simulink model "final_quadruped_080622_vel_level control"  (R2021a)
settings: Solver=ode15s  StartTime=0.0  StopTime=10  RelTol=1e-3  EnableMultiTasking=on
values from neighbouring files (symbols this model uses):
  foot_x = 8    [bipedparameters.m]    (also in fcn.m; finalrobotParameters.m; finalrobotParameters_110522.m; finalrobotParameters_140522.m)
  foot_y = 6    [bipedparameters.m]    (also in fcn.m; finalrobotParameters.m; finalrobotParameters_110522.m; finalrobotParameters_140522.m)
  foot_z = 1    [bipedparameters.m]    (also in fcn.m; finalrobotParameters.m; finalrobotParameters_110522.m; finalrobotParameters_140522.m)
  height_plane = 0.025    [bipedparameters.m]    (also in finalrobotParameters.m; finalrobotParameters_110522.m; finalrobotParameters_140522.m; finalrobotParameters_240522.m)
  kd = 1000    [bipedparameters.m]    (also in finalrobotParameters_140522.m = 5; finalrobotParameters_240522.m)
  ki = 1000    [bipedparameters.m]    (also in finalrobotParameters_140522.m = 5; finalrobotParameters_240522.m)
  kp = 1000    [bipedparameters.m]    (also in finalrobotParameters_140522.m = 5; finalrobotParameters_240522.m)
  lower_leg_length = 10    [bipedparameters.m]    (also in fcn.m; finalrobotParameters.m; finalrobotParameters_110522.m; finalrobotParameters_140522.m)
  m_ll = density*leg_radius*leg_radius*lower_leg_length*3.141592653589*0.01*0.01*0.01    (= 0.0176714586764)    [bipedparameters.m]    (also in fcn.m; finalrobotParameters_140522.m; finalrobotParameters_240522.m; hdotlb.m)
  m_ul = density*leg_radius*leg_radius*upper_leg_length*3.141592653589*0.01*0.01*0.01    (= 0.0176714586764)    [bipedparameters.m]    (also in fcn.m; finalrobotParameters_140522.m; finalrobotParameters_240522.m; hdotlb.m)
  plane_x = 25    [bipedparameters.m]    (also in finalrobotParameters.m; finalrobotParameters_110522.m; finalrobotParameters_140522.m; finalrobotParameters_240522.m)
  plane_y = 3    [bipedparameters.m]    (also in finalrobotParameters.m; finalrobotParameters_110522.m; finalrobotParameters_140522.m; finalrobotParameters_240522.m)
  torso_offset_x = -0.5    [bipedparameters.m]    (also in finalrobotParameters.m = 10; finalrobotParameters_110522.m = 10; finalrobotParameters_140522.m = 10; finalrobotParameters_240522.m = 10)
  torso_offset_z = -2    [bipedparameters.m]    (also in finalrobotParameters.m; finalrobotParameters_110522.m; finalrobotParameters_140522.m; finalrobotParameters_240522.m)
  torso_x = 5    [bipedparameters.m]    (also in fcn.m = 25; finalrobotParameters.m = 25; finalrobotParameters_110522.m = 25; finalrobotParameters_140522.m = 25)
  torso_y = 10    [bipedparameters.m]    (also in fcn.m = 16; finalrobotParameters.m = 16; finalrobotParameters_110522.m = 16; finalrobotParameters_140522.m = 16)
  torso_z = 8    [bipedparameters.m]    (also in fcn.m = 10; finalrobotParameters.m = 10; finalrobotParameters_110522.m = 10; finalrobotParameters_140522.m = 10)
  upper_leg_length = 10    [bipedparameters.m]    (also in fcn.m; finalrobotParameters.m; finalrobotParameters_110522.m; finalrobotParameters_140522.m)
undefined symbols (not defined in the file or in its folder): angleLFknee, speedLFknee, torqueLFknee, X, Y, Z
libraries: nesl_utility x105, sm_lib x71, Contact_Forces_Lib x16, pid_lib x12, fl_lib x3
(part 1 of 6)
settings Model: Creator=Durbadal Guest  LastModifiedBy=Saniya
settings SolverCC: AlgebraicLoopSolver=TrustRegion
settings DataIOCC: LimitDataPoints=on  SaveFormat=StructureWithTime  ReturnWorkspaceOutputs=off
settings OptimizationCC: LifeSpan=inf
settings DebuggingCC: SFUnexpectedBacktrackingDiag=warning  SFNoUnconditionalDefaultTransitionDiag=warning  SFExecutionAtInitializationDiag=none  SFMachineParentedDataDiag=warning  ArithmeticOperatorsInVariantConditions=warning
settings HardwareCC: ProdBitPerSizeT=32  ProdBitPerPtrDiffT=32  ProdWordSize=32  ProdHWDeviceType=Specified
settings SFSimCC: SimUseLocalCustomCode=off  CustomCodeUndefinedFunction=UseInterfaceOnly
settings RTWCC: RTWUseLocalCustomCode=off
settings CodeAppCC: StateflowObjectComments=on
settings GRTTargetCC: TargetLangStandard=C89/C90 (ANSI)
settings ConfigComp: CovMetricSettings=dw  CovSaveCumulativeToWorkspaceVar=on  CovSaveSingleToWorkspaceVar=on  CovExternalEMLEnable=off  CovSFcnEnable=off
settings SimscapeCC: SimscapeNominalValues="[{\"value\":\"10\",\"unit\":\"V\"},{\"value\":\"1\",\"unit\":\"A\"},{\"value\":\"10\",\"unit\":\"N*m\"},{\"value\":\"10\",\"unit\":\"bar\"},{\"value\":\"100\",\"unit\":\"kJ/kg\"},{\"value\":\"1\",\"unit\":\"kW\"},{\"value\":\"300\",\"unit\":\"K\"},{\"value\":\"100\",\"unit\":\"cm^3/s\"},{\"value\":\"1\",\"unit\":\"kN\"},{\"value\":\"1\",\"unit\":\"g/cm^3\"},{\"value\":\"1\",\"unit\":\"l\"},{\"value\":\"1\",\"unit\":\"cm^2\"},{\"value\":\"60\",\"unit\":\"Hz\"}]"  SimscapeLogType=all  SimscapeLogDataHistory=10000
settings ConfigurationSet: Description=SimMechanics 2G
settings DiagnosticsConfigSet: SimMechanicsRigidlyBoundBlock=none

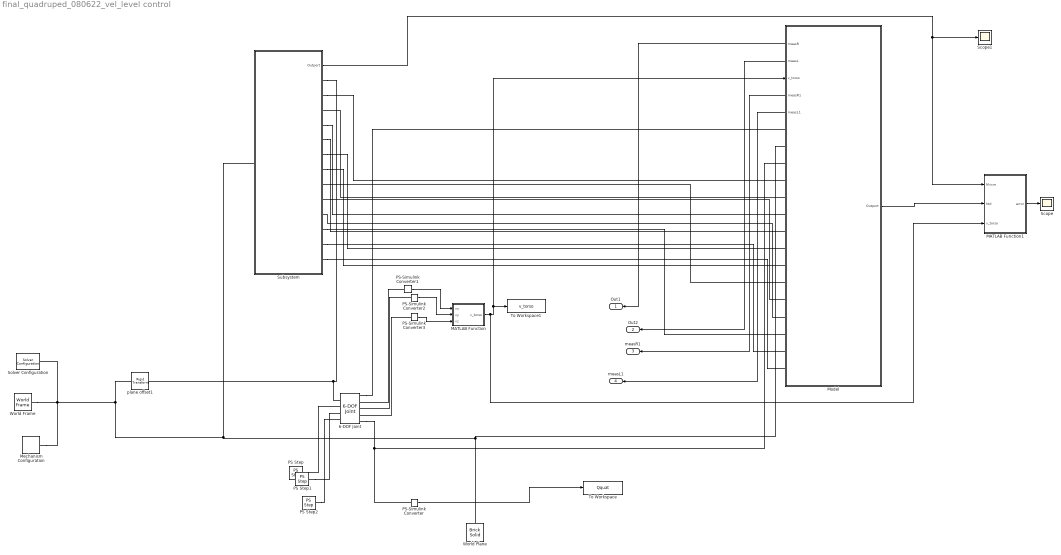
== system final_quadruped_080622_vel_level control ==
  6-DOF Joint : sm_lib/Joints/6-DOF Joint  JointMode=Normal  SenseConstraintForce=off  SenseConstraintForceX=off  SenseConstraintForceY=off  SenseConstraintForceZ=off  SenseConstraintTorque=off  SenseConstraintTorqueX=off  SenseConstraintTorqueY=off  SenseConstraintTorqueZ=off  SenseTotalForce=off  SenseTotalForceX=off  SenseTotalForceY=off  SenseTotalForceZ=off  SenseTotalTorque=off  SenseTotalTorqueX=off  SenseTotalTorqueY=off  SenseTotalTorqueZ=off  CompositeWrenchDir=FollowerOnBase  CompositeWrenchFrame=BaseFrame  PxEquilibriumPosition=0  PxEquilibriumPositionUnits=m  PxSpringStiffness=0  PxSpringStiffnessUnits=N/m  PxDampingCoefficient=0  PxDampingCoefficientUnits=N/(m/s)  PxTorqueActuationMode=InputTorque  PxMotionActuationMode=ComputedMotion  PxSensePosition=off  PxSenseVelocity=on  PxSenseAcceleration=off  PxSenseTorqueForce=off  PxSenseLowerLimitTorqueForce=off  PxSenseUpperLimitTorqueForce=off  PxLowerLimitSpecify=off  PxLowerLimitBound=-1  PxLowerLimitBoundUnits=m  PxLowerLimitStiffness=1e6  PxLowerLimitStiffnessUnits=N/m  PxLowerLimitDamping=1e3  PxLowerLimitDampingUnits=N/(m/s)  PxLowerLimitTransitionRegionWidth=1e-4  PxLowerLimitTransitionRegionWidthUnits=m  PxUpperLimitSpecify=off  PxUpperLimitBound=1  PxUpperLimitBoundUnits=m  PxUpperLimitStiffness=1e6  PxUpperLimitStiffnessUnits=N/m  PxUpperLimitDamping=1e3  PxUpperLimitDampingUnits=N/(m/s)  PxUpperLimitTransitionRegionWidth=1e-4  PxUpperLimitTransitionRegionWidthUnits=m  PxPositionTargetSpecify=on  PxPositionTargetPriority=High  PxPositionTargetValue=0  PxPositionTargetValueUnits=m  PxVelocityTargetSpecify=off  PxVelocityTargetPriority=High  PxVelocityTargetValue=0  PxVelocityTargetValueUnits=m/s  PyEquilibriumPosition=0  PyEquilibriumPositionUnits=m  PySpringStiffness=0  PySpringStiffnessUnits=N/m  PyDampingCoefficient=0  PyDampingCoefficientUnits=N/(m/s)  PyTorqueActuationMode=InputTorque  PyMotionActuationMode=ComputedMotion  PySensePosition=off  PySenseVelocity=on  PySenseAcceleration=off  PySenseTorqueForce=off  PySenseLowerLimitTorqueForce=off  PySenseUpperLimitTorqueForce=off  PyLowerLimitSpecify=off  PyLowerLimitBound=-1  PyLowerLimitBoundUnits=m  PyLowerLimitStiffness=1e6  PyLowerLimitStiffnessUnits=N/m  PyLowerLimitDamping=1e3  PyLowerLimitDampingUnits=N/(m/s)  PyLowerLimitTransitionRegionWidth=1e-4  PyLowerLimitTransitionRegionWidthUnits=m  PyUpperLimitSpecify=off  PyUpperLimitBound=1  PyUpperLimitBoundUnits=m  PyUpperLimitStiffness=1e6  PyUpperLimitStiffnessUnits=N/m  PyUpperLimitDamping=1e3  PyUpperLimitDampingUnits=N/(m/s)  PyUpperLimitTransitionRegionWidth=1e-4  PyUpperLimitTransitionRegionWidthUnits=m  PyPositionTargetSpecify=on  PyPositionTargetPriority=High  PyPositionTargetValue=0  PyPositionTargetValueUnits=m  PyVelocityTargetSpecify=off  PyVelocityTargetPriority=High  PyVelocityTargetValue=0  PyVelocityTargetValueUnits=m/s  PzEquilibriumPosition=0  PzEquilibriumPositionUnits=m  PzSpringStiffness=0  PzSpringStiffnessUnits=N/m  PzDampingCoefficient=0  PzDampingCoefficientUnits=N/(m/s)  PzTorqueActuationMode=InputTorque  PzMotionActuationMode=ComputedMotion  PzSensePosition=off  PzSenseVelocity=on  PzSenseAcceleration=off  PzSenseTorqueForce=off  PzSenseLowerLimitTorqueForce=off  PzSenseUpperLimitTorqueForce=off  PzLowerLimitSpecify=off  PzLowerLimitBound=-1  PzLowerLimitBoundUnits=m  PzLowerLimitStiffness=1e6  PzLowerLimitStiffnessUnits=N/m  PzLowerLimitDamping=1e3  PzLowerLimitDampingUnits=N/(m/s)  PzLowerLimitTransitionRegionWidth=1e-4  PzLowerLimitTransitionRegionWidthUnits=m  PzUpperLimitSpecify=off  PzUpperLimitBound=1  PzUpperLimitBoundUnits=m  PzUpperLimitStiffness=1e6  PzUpperLimitStiffnessUnits=N/m  PzUpperLimitDamping=1e3  PzUpperLimitDampingUnits=N/(m/s)  PzUpperLimitTransitionRegionWidth=1e-4  PzUpperLimitTransitionRegionWidthUnits=m  PzPositionTargetSpecify=on  PzPositionTargetPriority=High  PzPositionTargetValue=0  PzPositionTargetValueUnits=m  PzVelocityTargetSpecify=off  PzVelocityTargetPriority=High  PzVelocityTargetValue=0  PzVelocityTargetValueUnits=m/s  SphDefPosRotationMethod=None  SphDefPosRotationAngleUnits=deg  SphDefPosRotationStandardAxis=+Z  SphDefPosRotationAngle=0.0  SphDefPosRotationArbitraryAxis=[0 0 1]  SphDefPosFollAlignAxisA=+X  SphDefPosBaseAlignAxisA=+Y  SphDefPosFollAlignAxisB=+Y  SphDefPosBaseAlignAxisB=+Z  SphDefPosRotationSequenceAxes=FollowerAxes  SphDefPosRotationSequence=XYX  SphDefPosRotationSequenceAngles=[0 0 0]  SphDefPosRotationSequenceAnglesUnits=deg  SphDefPosRotationMatrix=[1 0 0; 0 1 0; 0 0 1]  SphEqPosRotationMethod=None  SphEqPosRotationAngleUnits=deg  SphEqPosRotationStandardAxis=+Z  SphEqPosRotationAngle=0.0  SphEqPosRotationArbitraryAxis=[0 0 1]  SphEqPosFollAlignAxisA=+X  SphEqPosBaseAlignAxisA=+Y  SphEqPosFollAlignAxisB=+Y  SphEqPosBaseAlignAxisB=+Z  SphEqPosRotationSequenceAxes=FollowerAxes  SphEqPosRotationSequence=XYX  SphEqPosRotationSequenceAngles=[0 0 0]  SphEqPosRotationSequenceAnglesUnits=deg  SphEqPosRotationMatrix=[1 0 0; 0 1 0; 0 0 1]  SphSpringStiffness=0  SphSpringStiffnessUnits=N*m/deg  SphDampingCoefficient=world_rot_damping  SphDampingCoefficientUnits=N*m/(deg/s)  SphActuateTorqueX=off  SphActuateTorqueY=off  SphActuateTorqueZ=off  SphActuateTorque=off  SphTorqueActuationMode=NoTorque  SphMotionActuationMode=ComputedMotion  SphActuationFrame=BaseFrame  SphSensePosition=on  SphSenseVelocityX=off  SphSenseVelocityY=off  SphSenseVelocityZ=off  SphSenseVelocity=off  SphSenseAccelerationX=off  SphSenseAccelerationY=off  SphSenseAccelerationZ=off  SphSenseAcceleration=off  SphSenseTorqueX=off  SphSenseTorqueY=off  SphSenseTorqueZ=off  SphSenseTorqueForce=off  SphSenseLowerLimitTorqueMag=off  SphSenseUpperLimitTorqueMag=off  SphSensingFrame=BaseFrame  SphLowerLimitSpecify=off  SphLowerLimitBound=15  SphLowerLimitBoundUnits=deg  SphLowerLimitStiffness=1e4  SphLowerLimitStiffnessUnits=N*m/deg  SphLowerLimitDamping=10  SphLowerLimitDampingUnits=N*m/(deg/s)  SphLowerLimitTransitionRegionWidth=0.1  SphLowerLimitTransitionRegionWidthUnits=deg  SphUpperLimitSpecify=off  SphUpperLimitBound=45  SphUpperLimitBoundUnits=deg  SphUpperLimitStiffness=1e4  SphUpperLimitStiffnessUnits=N*m/deg  SphUpperLimitDamping=10  SphUpperLimitDampingUnits=N*m/(deg/s)  SphUpperLimitTransitionRegionWidth=0.1  SphUpperLimitTransitionRegionWidthUnits=deg  SphPositionTargetRotationMethod=None  SphPositionTargetRotationAngleUnits=deg  SphPositionTargetRotationStandardAxis=+Z  SphPositionTargetRotationAngle=0.0  SphPositionTargetRotationArbitraryAxis=[0 0 1]  SphPositionTargetFollAlignAxisA=+X  SphPositionTargetBaseAlignAxisA=+Y  SphPositionTargetFollAlignAxisB=+Y  SphPositionTargetBaseAlignAxisB=+Z  SphPositionTargetRotationSequenceAxes=FollowerAxes  SphPositionTargetRotationSequence=XYX  SphPositionTargetRotationSequenceAngles=[0 0 0]  SphPositionTargetRotationSequenceAnglesUnits=deg  SphPositionTargetRotationMatrix=[1 0 0; 0 1 0; 0 0 1]  SphPositionTargetSpecify=off  SphPositionTargetPriority=High  SphVelocityTargetValue=[0 0 0]  SphVelocityTargetValueUnits=deg/s  SphVelocityTargetSpecify=off  SphVelocityTargetPriority=High  SphVelocityTargetInFollowerFrame=on
  MATLAB Function : MATLAB Function  TreatAsAtomicUnit=on
  MATLAB Function1 : MATLAB Function  TreatAsAtomicUnit=on
  Mechanism Configuration : sm_lib/Utilities/Mechanism Configuration  UniformGravity=Constant  GravityVector=[0 0 -9.80665]  GravityVectorUnits=m/s^2  GravityUnits=m/s^2  LinearizationDelta=0.001  JointModeTransitionNonlinearIterations=2
  Model : Subsystem
      settings: PortSchema="{\"entries\":[{\"content\":{\"sides\":[{\"content\":{\"connectorIds\":[\"Out5\"]},\"type\":\"ConnectorPlacement.EquallySpacedRectSide\",\"uuid\":\"648e0f1c-94fd-432d-b314-f859853b28dc\"},{\"content\":{\"connectorIds\":[\"Out1\",\"Out2\",\"In1\",\"Out3\",\"Out4\",\"RConn1\",\"RConn2\",\"RConn3\",\"RConn4\",\"RConn5\",\"RConn6\",\"RConn7\",\"RConn8\",\"RConn9\",\"RConn10\",\"RConn11\",\"RConn12\",\"RConn13\",\"RConn14\",\"RConn15\"],\"side\":\"RIGHT\"},\"type\":\"ConnectorPlacement.EquallySpacedRectSide\",\"uuid\":\"4a085109-6c7b-452e-9c34-33db191f9143\"},{\"content\":{\"connectorIds\":[],\"side\":\"TOP\"},\"type\":\"ConnectorPlacement.EquallySpacedRectSide\",\"uuid\":\"a578f37e-fb06-4d5d-8e21-8bc1ba433708\"}]},\"type\":\"ConnectorPlacement.EquallySpacedConnector\",\"uuid\":\"512c293d-fddc-4597-a716-0ff05cc0aa2f\"}],\"packageUris\":[\"http://schema.mathworks.com/mf0/Connector/R2020b\"],\"version\":\"1.0\"}"
  PS Step : fl_lib/Physical Signals/Sources/PS Step  step_time=0 s  initial_value=0 N  final_value=1 N
      settings: SourceProductBaseCode=SS
  PS Step1 : fl_lib/Physical Signals/Sources/PS Step  step_time=0 s  initial_value=0 N  final_value=0 N
      settings: SourceProductBaseCode=SS
  PS Step2 : fl_lib/Physical Signals/Sources/PS Step  step_time=0 s  initial_value=0 N  final_value=5 N
      settings: SourceProductBaseCode=SS
  PS-Simulink Converter{,1..3} (4 alike) : nesl_utility/PS-Simulink Converter  PhysicalDomain=network_engine_domain  SubClassName=ps_output  LeftPortType=input  RightPortType=output  PseudoPeriodic=off  Frequencies=[]  Unit=inherit  AffineConversion=off
      settings: SourceProductBaseCode=PW,SS
  Scope : Scope
  Scope1 : Scope
  Solver Configuration : nesl_utility/Solver Configuration  PhysicalDomain=network_engine_domain  SubClassName=solver  LeftPortType=input  RightPortType=generic  Tones=[]  Harmonics=[]  SimulateNoise=off  Profile=off  UseLocalSampling=off  EnableSwitchedLinearOptims=on  FrequencyDomain=off  UseCCode=off  RelTol=0.001  AbsTol=1e-06  MinStep=1e-09  ToWorkspace=off  RevertToSquareIcSolve=off  NumHomotopyIterations=100  PhasorMode=off  PhasorModeNumHarmonics=1  DoDC=off  ResidualTolerance=1e-09  UseLocalSolver=off  LocalSolverChoice=NE_BACKWARD_EULER_ADVANCER  LocalSolverSampleTime=0.001  DoFixedCost=off  MaxNonlinIter=3  MaxModeIter=2  ComputeImpulses=off  ImpulseIterations=2  LinearAlgebra=Full  EquationFormulation=NE_TIME_EF  DelaysMemoryBudget=1024  AutomaticFiltering=on  FilteringTimeConstant=0.001  PartitionStorageMethod=AS_NEEDED  PartitionMemoryBudget=1024  PartitionMethod=FAST
      settings: SourceProductBaseCode=PW,SS
  Subsystem : Subsystem
  To Workspace : ToWorkspace  VariableName=Qquat  SaveFormat=Timeseries  SampleTime=-1
  To Workspace1 : ToWorkspace  VariableName=v_torso  SaveFormat=Timeseries  SampleTime=-1
  World Frame : sm_lib/Frames and Transforms/World Frame
  World Plane : sm_lib/Body Elements/Brick Solid  GraphicAmbientColor=[0.15 0.15 0.15 1.0]  BasedOnType=Density  BrickDimensions=[plane_x plane_y height_plane]  BrickDimensionUnits=m  CenterOfMass=[0 0 0]  CenterOfMassUnits=m  GraphicDiffuseColor=[1.0 0.2 0.2]  Density=2000  DensityUnits=kg/m^3  DoExposeReferenceFrame=on  GraphicEmissiveColor=[0.0 0.0 0.0 1.0]  ExportEntireGeometry=off  SerializedFrames=<Frames/>  MarkerShape=Sphere  MarkerSize=10  GraphicType=FromGeometry  InertiaType=CalculateFromGeometry  Mass=1  MassUnits=kg  MomentsOfInertia=[1 1 1]  MomentsOfInertiaUnits=kg*m^2  GraphicOpacity=1.0  ProductsOfInertia=[1 1 1]  ProductsOfInertiaUnits=kg*m^2  GraphicShininess=75  GraphicSpecularColor=[0.5 0.5 0.5 1.0]  GraphicVisPropType=SimpleVisualProperties
  plane offset1 : sm_lib/Frames and Transforms/Rigid Transform  TranslationMethod=StandardAxis  TranslationStandardOffset=24.1  TranslationLengthUnit=cm  TranslationStandardAxis=+Z  TranslationCartesianOffset=[0 0 0]  TranslationROffset=0  TranslationROffsetUnits=m  TranslationZOffset=0  TranslationZOffsetUnits=m  TranslationThetaOffset=0  TranslationThetaOffsetUnits=deg  RotationMethod=None  RotationAngleUnits=deg  RotationStandardAxis=+Z  RotationAngle=0.0  RotationArbitraryAxis=[0 0 1]  FollAlignAxisA=+X  BaseAlignAxisA=+Y  FollAlignAxisB=+Y  BaseAlignAxisB=+Z  RotationSequenceAxes=FollowerAxes  RotationSequence=XYX  RotationSequenceAngles=[0 0 0]  RotationSequenceAnglesUnits=deg  RotationMatrix=[1 0 0; 0 1 0; 0 0 1]
  Out1 : Outport  VectorParamsAs1DForOutWhenUnconnected=off
  Out2 : Outport  Port=2  VectorParamsAs1DForOutWhenUnconnected=off
  measR1 : Outport  Port=3  VectorParamsAs1DForOutWhenUnconnected=off
  measL1 : Outport  Port=4  VectorParamsAs1DForOutWhenUnconnected=off
  wires:
  Model/1(measR) -> Out1/1
  Model/2(measL) -> Out2/1
  Model/3(measR1) -> measR1/1
  Model/4(measL1) -> measL1/1
  PS-Simulink Converter/1 -> To Workspace/1
  PS-Simulink Converter1/1 -> MATLAB Function/1(vx)
  PS-Simulink Converter2/1 -> MATLAB Function/2(vy)
  PS-Simulink Converter3/1 -> MATLAB Function/3(vz)
  MATLAB Function/1(v_torso) -> MATLAB Function1/3(v_torso), To Workspace1/1, Model/1(v_torso)
  Subsystem/1(Outport) -> Scope1/1, MATLAB Function1/1(Mvcm)
  Model/5(Outport) -> MATLAB Function1/2(htd)
  MATLAB Function1/1(error) -> Scope/1
  connections:
  6-DOF Joint/RConn1 -- Model/RConn1
  6-DOF Joint/LConn1 -- plane offset1/RConn1 -- Subsystem/RConn1
  6-DOF Joint/RConn5 -- PS-Simulink Converter/LConn1 -- Model/RConn3
  PS-Simulink Converter1/LConn1 -- 6-DOF Joint/RConn2
  PS-Simulink Converter2/LConn1 -- 6-DOF Joint/RConn3
  PS-Simulink Converter3/LConn1 -- 6-DOF Joint/RConn4
  plane offset1/LConn1 -- Solver Configuration/RConn1 -- World Frame/RConn1 -- Mechanism Configuration/RConn1 -- World Plane/RConn1 -- Model/RConn2 -- Subsystem/LConn1
  Subsystem/RConn2 -- Model/RConn4
  Model/RConn5 -- Subsystem/RConn3
  Subsystem/RConn4 -- Model/RConn6
  Subsystem/RConn5 -- Model/RConn7
  Subsystem/RConn6 -- Model/RConn8
  Subsystem/RConn7 -- Model/RConn9
  Model/RConn10 -- Subsystem/RConn8
  Model/RConn11 -- Subsystem/RConn9
  Model/RConn12 -- Subsystem/RConn10
  Subsystem/RConn11 -- Model/RConn13
  Subsystem/RConn12 -- Model/RConn14
  Subsystem/RConn13 -- Model/RConn15
  6-DOF Joint/LConn2 -- PS Step/RConn1
  PS Step1/RConn1 -- 6-DOF Joint/LConn3
  PS Step2/RConn1 -- 6-DOF Joint/LConn4

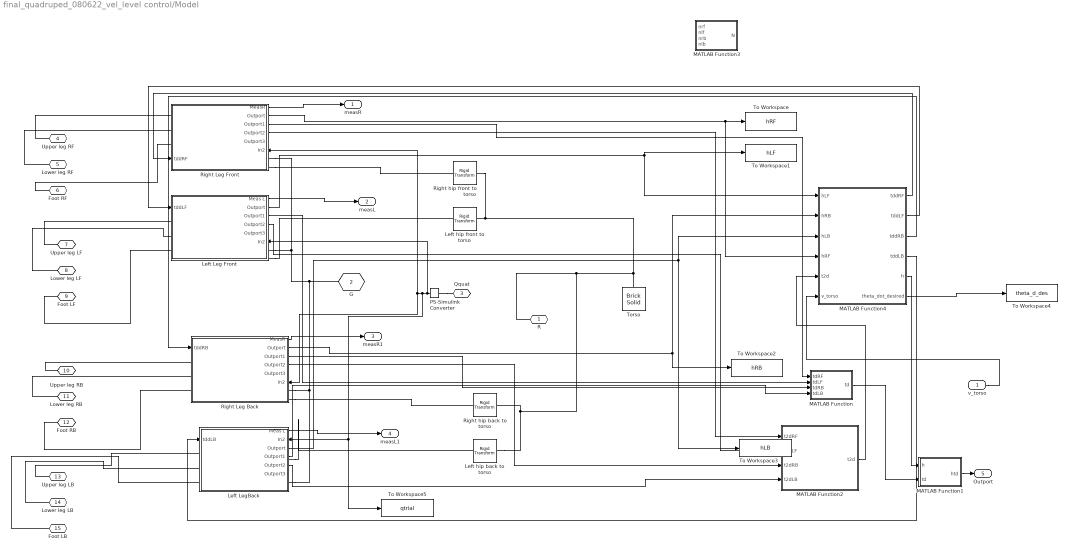
== system final_quadruped_080622_vel_level control/Model ==
  v_torso : Inport
  Left Leg Front : Subsystem
      settings: PortSchema="{\"entries\":[{\"content\":{\"sides\":[{\"content\":{\"connectorIds\":[\"In1\",\"LConn1\",\"LConn2\",\"LConn3\"]},\"type\":\"ConnectorPlacement.EquallySpacedRectSide\",\"uuid\":\"1507813e-36a9-49af-9b0a-e3846bbe4283\"},{\"content\":{\"connectorIds\":[\"Out1\",\"Out2\",\"Out3\",\"Out4\",\"Out5\",\"In2\",\"RConn1\",\"RConn2\"],\"side\":\"RIGHT\"},\"type\":\"ConnectorPlacement.EquallySpacedRectSide\",\"uuid\":\"5066f35d-c1fd-4314-a197-bec554758284\"},{\"content\":{\"connectorIds\":[],\"side\":\"TOP\"},\"type\":\"ConnectorPlacement.EquallySpacedRectSide\",\"uuid\":\"2e06378b-9fb7-4b7b-9b3c-942eabd1dde3\"}]},\"type\":\"ConnectorPlacement.EquallySpacedConnector\",\"uuid\":\"ce1b660b-7838-4ff4-b715-b13e7b6fd161\"}],\"packageUris\":[\"http://schema.mathworks.com/mf0/Connector/R2020b\"],\"version\":\"1.0\"}"
  Left LegBack : Subsystem
      settings: PortSchema="{\"entries\":[{\"content\":{\"sides\":[{\"content\":{\"connectorIds\":[\"In1\",\"LConn1\",\"LConn2\",\"LConn3\"]},\"type\":\"ConnectorPlacement.EquallySpacedRectSide\",\"uuid\":\"22ee734e-d516-4767-9dd7-a84a6d7499a1\"},{\"content\":{\"connectorIds\":[\"Out1\",\"In2\",\"Out2\",\"Out3\",\"Out4\",\"Out5\",\"RConn1\",\"RConn2\"],\"side\":\"RIGHT\"},\"type\":\"ConnectorPlacement.EquallySpacedRectSide\",\"uuid\":\"10c942f7-94ea-46a3-ba7f-65e81ae36ff4\"},{\"content\":{\"connectorIds\":[],\"side\":\"TOP\"},\"type\":\"ConnectorPlacement.EquallySpacedRectSide\",\"uuid\":\"f15406a8-c456-4a24-8e06-fd295582a32c\"}]},\"type\":\"ConnectorPlacement.EquallySpacedConnector\",\"uuid\":\"8882591f-f267-4868-b883-a2707b6c50ed\"}],\"packageUris\":[\"http://schema.mathworks.com/mf0/Connector/R2020b\"],\"version\":\"1.0\"}"
  Left hip back to torso : sm_lib/Frames and Transforms/Rigid Transform  TranslationMethod=Cartesian  TranslationStandardOffset=0  TranslationLengthUnit=cm  TranslationStandardAxis=+Z  TranslationCartesianOffset=[-torso_offset_x torso_y/2 torso_offset_z]  TranslationROffset=0  TranslationROffsetUnits=m  TranslationZOffset=0  TranslationZOffsetUnits=m  TranslationThetaOffset=0  TranslationThetaOffsetUnits=deg  RotationMethod=None  RotationAngleUnits=deg  RotationStandardAxis=+Z  RotationAngle=0.0  RotationArbitraryAxis=[0 0 1]  FollAlignAxisA=+X  BaseAlignAxisA=+Y  FollAlignAxisB=+Y  BaseAlignAxisB=+Z  RotationSequenceAxes=FollowerAxes  RotationSequence=XYX  RotationSequenceAngles=[0 0 0]  RotationSequenceAnglesUnits=deg  RotationMatrix=[1 0 0; 0 1 0; 0 0 1]
  Left hip front to torso : sm_lib/Frames and Transforms/Rigid Transform  TranslationMethod=Cartesian  TranslationStandardOffset=0  TranslationLengthUnit=cm  TranslationStandardAxis=+Z  TranslationCartesianOffset=[torso_offset_x torso_y/2 torso_offset_z]  TranslationROffset=0  TranslationROffsetUnits=m  TranslationZOffset=0  TranslationZOffsetUnits=m  TranslationThetaOffset=0  TranslationThetaOffsetUnits=deg  RotationMethod=None  RotationAngleUnits=deg  RotationStandardAxis=+Z  RotationAngle=0.0  RotationArbitraryAxis=[0 0 1]  FollAlignAxisA=+X  BaseAlignAxisA=+Y  FollAlignAxisB=+Y  BaseAlignAxisB=+Z  RotationSequenceAxes=FollowerAxes  RotationSequence=XYX  RotationSequenceAngles=[0 0 0]  RotationSequenceAnglesUnits=deg  RotationMatrix=[1 0 0; 0 1 0; 0 0 1]
  MATLAB Function : MATLAB Function  TreatAsAtomicUnit=on
  MATLAB Function1 : MATLAB Function  TreatAsAtomicUnit=on
  MATLAB Function2 : MATLAB Function  TreatAsAtomicUnit=on
  MATLAB Function3 : MATLAB Function  TreatAsAtomicUnit=on
  MATLAB Function4 : MATLAB Function  TreatAsAtomicUnit=on
  PS-Simulink Converter : nesl_utility/PS-Simulink Converter  PhysicalDomain=network_engine_domain  SubClassName=ps_output  LeftPortType=input  RightPortType=output  PseudoPeriodic=off  Frequencies=[]  Unit=inherit  AffineConversion=off
      settings: SourceProductBaseCode=PW,SS
  Right Leg Back : Subsystem
      settings: PortSchema="{\"entries\":[{\"content\":{\"sides\":[{\"content\":{\"connectorIds\":[\"In1\",\"LConn1\",\"LConn2\",\"LConn3\"]},\"type\":\"ConnectorPlacement.EquallySpacedRectSide\",\"uuid\":\"22ee734e-d516-4767-9dd7-a84a6d7499a1\"},{\"content\":{\"connectorIds\":[\"Out1\",\"Out2\",\"Out3\",\"Out4\",\"Out5\",\"In2\",\"RConn1\",\"RConn2\"],\"side\":\"RIGHT\"},\"type\":\"ConnectorPlacement.EquallySpacedRectSide\",\"uuid\":\"10c942f7-94ea-46a3-ba7f-65e81ae36ff4\"},{\"content\":{\"connectorIds\":[],\"side\":\"TOP\"},\"type\":\"ConnectorPlacement.EquallySpacedRectSide\",\"uuid\":\"f15406a8-c456-4a24-8e06-fd295582a32c\"}]},\"type\":\"ConnectorPlacement.EquallySpacedConnector\",\"uuid\":\"8882591f-f267-4868-b883-a2707b6c50ed\"}],\"packageUris\":[\"http://schema.mathworks.com/mf0/Connector/R2020b\"],\"version\":\"1.0\"}"
  "Right Leg Front " : Subsystem
      settings: PortSchema="{\"entries\":[{\"content\":{\"sides\":[{\"content\":{\"connectorIds\":[\"LConn1\",\"LConn2\",\"LConn3\",\"In1\"]},\"type\":\"ConnectorPlacement.EquallySpacedRectSide\",\"uuid\":\"22ee734e-d516-4767-9dd7-a84a6d7499a1\"},{\"content\":{\"connectorIds\":[\"Out1\",\"Out2\",\"Out3\",\"Out4\",\"Out5\",\"In2\",\"RConn1\",\"RConn2\"],\"side\":\"RIGHT\"},\"type\":\"ConnectorPlacement.EquallySpacedRectSide\",\"uuid\":\"10c942f7-94ea-46a3-ba7f-65e81ae36ff4\"},{\"content\":{\"connectorIds\":[],\"side\":\"TOP\"},\"type\":\"ConnectorPlacement.EquallySpacedRectSide\",\"uuid\":\"f15406a8-c456-4a24-8e06-fd295582a32c\"}]},\"type\":\"ConnectorPlacement.EquallySpacedConnector\",\"uuid\":\"8882591f-f267-4868-b883-a2707b6c50ed\"}],\"packageUris\":[\"http://schema.mathworks.com/mf0/Connector/R2020b\"],\"version\":\"1.0\"}"
  Right hip back to torso : sm_lib/Frames and Transforms/Rigid Transform  TranslationMethod=Cartesian  TranslationStandardOffset=0  TranslationLengthUnit=cm  TranslationStandardAxis=+Z  TranslationCartesianOffset=[-torso_offset_x -torso_y/2 torso_offset_z]  TranslationROffset=0  TranslationROffsetUnits=m  TranslationZOffset=0  TranslationZOffsetUnits=m  TranslationThetaOffset=0  TranslationThetaOffsetUnits=deg  RotationMethod=None  RotationAngleUnits=deg  RotationStandardAxis=+Z  RotationAngle=0.0  RotationArbitraryAxis=[0 0 1]  FollAlignAxisA=+X  BaseAlignAxisA=+Y  FollAlignAxisB=+Y  BaseAlignAxisB=+Z  RotationSequenceAxes=FollowerAxes  RotationSequence=XYX  RotationSequenceAngles=[0 0 0]  RotationSequenceAnglesUnits=deg  RotationMatrix=[1 0 0; 0 1 0; 0 0 1]
  Right hip front to torso : sm_lib/Frames and Transforms/Rigid Transform  TranslationMethod=Cartesian  TranslationStandardOffset=0  TranslationLengthUnit=cm  TranslationStandardAxis=+Z  TranslationCartesianOffset=[torso_offset_x -torso_y/2 torso_offset_z]  TranslationROffset=0  TranslationROffsetUnits=m  TranslationZOffset=0  TranslationZOffsetUnits=m  TranslationThetaOffset=0  TranslationThetaOffsetUnits=deg  RotationMethod=None  RotationAngleUnits=deg  RotationStandardAxis=+Z  RotationAngle=0.0  RotationArbitraryAxis=[0 0 1]  FollAlignAxisA=+X  BaseAlignAxisA=+Y  FollAlignAxisB=+Y  BaseAlignAxisB=+Z  RotationSequenceAxes=FollowerAxes  RotationSequence=XYX  RotationSequenceAngles=[0 0 0]  RotationSequenceAnglesUnits=deg  RotationMatrix=[1 0 0; 0 1 0; 0 0 1]
  To Workspace : ToWorkspace  VariableName=hRF  SaveFormat=Timeseries  SampleTime=-1
  To Workspace1 : ToWorkspace  VariableName=hLF  SaveFormat=Timeseries  SampleTime=-1
  To Workspace2 : ToWorkspace  VariableName=hRB  SaveFormat=Timeseries  SampleTime=-1
  To Workspace3 : ToWorkspace  VariableName=hLB  SaveFormat=Timeseries  SampleTime=-1
  To Workspace4 : ToWorkspace  VariableName=theta_d_des  SaveFormat=Timeseries  SampleTime=-1
  To Workspace5 : ToWorkspace  VariableName=qtrial  SaveFormat=Timeseries  SampleTime=-1
  Torso : sm_lib/Body Elements/Brick Solid  GraphicAmbientColor=[0.15 0.15 0.15 1.0]  BasedOnType=Density  BrickDimensions=[torso_x torso_y torso_z]  BrickDimensionUnits=cm  CenterOfMass=[0 0 0]  CenterOfMassUnits=m  GraphicDiffuseColor=[0.5 0.5 0.5]  Density=1000  DensityUnits=kg/m^3  DoExposeReferenceFrame=on  GraphicEmissiveColor=[0.0 0.0 0.0 1.0]  ExportEntireGeometry=off  SerializedFrames=<Frames/>  MarkerShape=Sphere  MarkerSize=10  GraphicType=FromGeometry  InertiaType=CalculateFromGeometry  Mass=1  MassUnits=kg  MomentsOfInertia=[1 1 1]  MomentsOfInertiaUnits=kg*m^2  GraphicOpacity=1.0  ProductsOfInertia=[1 1 1]  ProductsOfInertiaUnits=kg*m^2  GraphicShininess=75  GraphicSpecularColor=[0.5 0.5 0.5 1.0]  GraphicVisPropType=SimpleVisualProperties
  R : PMIOPort  Side=Right
  G : PMIOPort  Port=2  Side=Right
  Qquat : PMIOPort  Port=3  Side=Right
  Upper leg RF : PMIOPort  Port=4  Side=Right
  Lower leg RF : PMIOPort  Port=5  Side=Right
  Foot RF : PMIOPort  Port=6  Side=Right
  Upper leg LF : PMIOPort  Port=7  Side=Right
  Lower leg LF : PMIOPort  Port=8  Side=Right
  Foot LF : PMIOPort  Port=9  Side=Right
  Upper leg RB : PMIOPort  Port=10  Side=Right
  Lower leg RB : PMIOPort  Port=11  Side=Right
  Foot RB : PMIOPort  Port=12  Side=Right
  Upper leg LB : PMIOPort  Port=13  Side=Right
  Lower leg LB : PMIOPort  Port=14  Side=Right
  Foot LB : PMIOPort  Port=15  Side=Right
  measR : Outport  VectorParamsAs1DForOutWhenUnconnected=off
  measL : Outport  Port=2  VectorParamsAs1DForOutWhenUnconnected=off
  measR1 : Outport  Port=3  VectorParamsAs1DForOutWhenUnconnected=off
  measL1 : Outport  Port=4  VectorParamsAs1DForOutWhenUnconnected=off
  Outport : Outport  Port=5
  wires:
  Left Leg Front/1("Meas L ") -> measL/1
  "Right Leg Front "/1(MeasR) -> measR/1
  Right Leg Back/1(MeasR) -> measR1/1
  Left LegBack/1("Meas L ") -> measL1/1
  "Right Leg Front "/2(Outport) -> MATLAB Function4/4(hRF), To Workspace/1
  Right Leg Back/2(Outport) -> To Workspace2/1, MATLAB Function4/2(hRB)
  Left LegBack/2(Outport) -> To Workspace3/1, MATLAB Function4/3(hLB)
  Left Leg Front/2(Outport) -> To Workspace1/1, MATLAB Function4/1(hLF)
  PS-Simulink Converter/1 -> "Right Leg Front "/2(In2), Right Leg Back/2(In2), To Workspace5/1, Left LegBack/2(In2), Left Leg Front/2(In2)
  v_torso/1 -> MATLAB Function4/6(v_torso)
  MATLAB Function4/1(tddRF) -> "Right Leg Front "/1(tddRF)
  MATLAB Function4/2(tddLF) -> Left Leg Front/1(tddLF)
  MATLAB Function4/3(tddRB) -> Right Leg Back/1(tddRB)
  MATLAB Function4/4(tddLB) -> Left LegBack/1(tddLB)
  "Right Leg Front "/3(Outport1) -> MATLAB Function/1(tdRF)
  Left Leg Front/3(Outport1) -> MATLAB Function/2(tdLF)
  Right Leg Back/3(Outport1) -> MATLAB Function/3(tdRB)
  Left LegBack/3(Outport1) -> MATLAB Function/4(tdLB)
  MATLAB Function4/5(h) -> MATLAB Function1/1(h)
  MATLAB Function/1(td) -> MATLAB Function1/2(td)
  MATLAB Function1/1(htd) -> Outport/1
  MATLAB Function4/6(theta_dot_desired) -> To Workspace4/1
  "Right Leg Front "/4(Outport2) -> MATLAB Function2/1(t2dRF)
  Left Leg Front/4(Outport2) -> MATLAB Function2/2(t2dLF)
  Right Leg Back/4(Outport2) -> MATLAB Function2/3(t2dRB)
  Left LegBack/4(Outport2) -> MATLAB Function2/4(t2dLB)
  MATLAB Function2/1(t2d) -> MATLAB Function4/5(t2d)
  connections:
  Left Leg Front/RConn2 -- Left hip front to torso/RConn1
  "Right Leg Front "/RConn2 -- Right hip front to torso/RConn1
  "Right Leg Front "/RConn1 -- Left Leg Front/RConn1 -- Left LegBack/RConn1 -- Right Leg Back/RConn1 -- G/RConn1
  Right Leg Back/RConn2 -- Right hip back to torso/RConn1
  Left LegBack/RConn2 -- Left hip back to torso/RConn1
  Right hip front to torso/LConn1 -- R/RConn1 -- Right hip back to torso/LConn1 -- Left hip back to torso/LConn1 -- Torso/RConn1 -- Left hip front to torso/LConn1
  PS-Simulink Converter/LConn1 -- Qquat/RConn1
  Upper leg RF/RConn1 -- "Right Leg Front "/LConn1
  Lower leg RF/RConn1 -- "Right Leg Front "/LConn2
  "Right Leg Front "/LConn3 -- Foot RF/RConn1
  Left Leg Front/LConn3 -- Foot LF/RConn1
  Left Leg Front/LConn1 -- Upper leg LF/RConn1
  Left Leg Front/LConn2 -- Lower leg LF/RConn1
  Upper leg RB/RConn1 -- Right Leg Back/LConn1
  Lower leg RB/RConn1 -- Right Leg Back/LConn2
  Foot RB/RConn1 -- Right Leg Back/LConn3
  Lower leg LB/RConn1 -- Left LegBack/LConn2
  Foot LB/RConn1 -- Left LegBack/LConn3
  Upper leg LB/RConn1 -- Left LegBack/LConn1

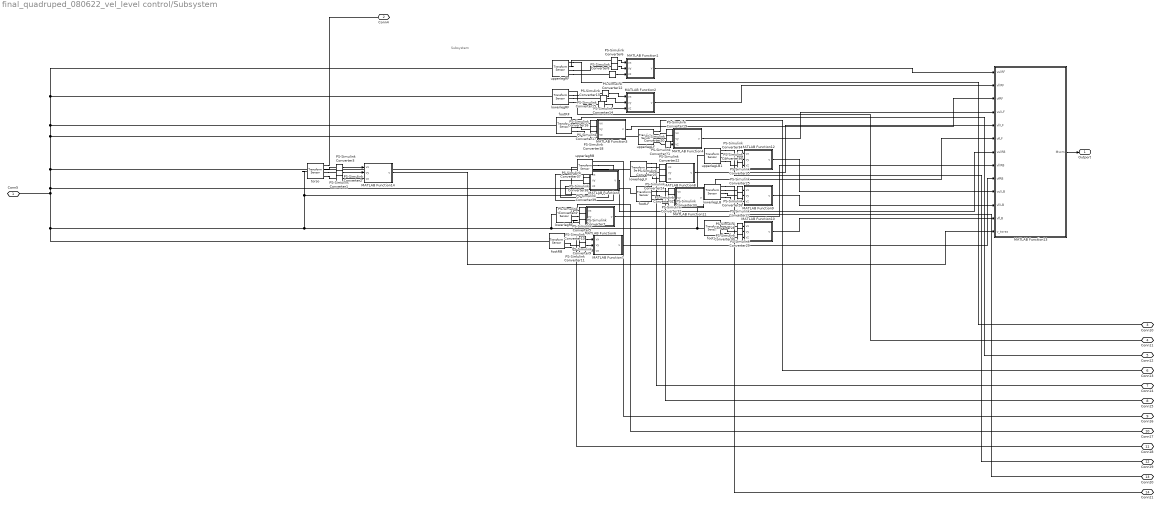
== system final_quadruped_080622_vel_level control/Subsystem ==
  note: Subsystem
  MATLAB Function1 : MATLAB Function  TreatAsAtomicUnit=on
  MATLAB Function10 : MATLAB Function  TreatAsAtomicUnit=on
  MATLAB Function11 : MATLAB Function  TreatAsAtomicUnit=on
  MATLAB Function12 : MATLAB Function  TreatAsAtomicUnit=on
  MATLAB Function13 : MATLAB Function  TreatAsAtomicUnit=on
  MATLAB Function14 : MATLAB Function  TreatAsAtomicUnit=on
  MATLAB Function2 : MATLAB Function  TreatAsAtomicUnit=on
  MATLAB Function3 : MATLAB Function  TreatAsAtomicUnit=on
  MATLAB Function4 : MATLAB Function  TreatAsAtomicUnit=on
  MATLAB Function5 : MATLAB Function  TreatAsAtomicUnit=on
  MATLAB Function6 : MATLAB Function  TreatAsAtomicUnit=on
  MATLAB Function7 : MATLAB Function  TreatAsAtomicUnit=on
  MATLAB Function8 : MATLAB Function  TreatAsAtomicUnit=on
  MATLAB Function9 : MATLAB Function  TreatAsAtomicUnit=on
  PS-Simulink Converter{1..39} (39 alike) : nesl_utility/PS-Simulink Converter  PhysicalDomain=network_engine_domain  SubClassName=ps_output  LeftPortType=input  RightPortType=output  PseudoPeriodic=off  Frequencies=[]  Unit=inherit  AffineConversion=off
      settings: SourceProductBaseCode=PW,SS
  footLB : sm_lib/Frames and Transforms/Transform Sensor  MeasurementFrame=World  SenseAngle=off  SenseAxis=off  SenseAngle1=off  SenseAngle2=off  SenseAngle3=off  SenseQ=off  SenseR=off  SenseOmegaX=off  SenseOmegaY=off  SenseOmegaZ=off  SenseOmega1=off  SenseOmega2=off  SenseOmega3=off  SenseQDot=off  SenseRDot=off  SenseAlphaX=off  SenseAlphaY=off  SenseAlphaZ=off  SenseAlpha1=off  SenseAlpha2=off  SenseAlpha3=off  SenseQDDot=off  SenseRDDot=off  SenseX=off  SenseY=off  SenseZ=off  SenseRad=off  SenseAzim=off  SenseDist=off  SenseInc=off  SenseXDot=on  SenseYDot=on  SenseZDot=on  SenseRadDot=off  SenseAzimDot=off  SenseDistDot=off  SenseIncDot=off  SenseXDDot=off  SenseYDDot=off  SenseZDDot=off  SenseRadDDot=off  SenseAzimDDot=off  SenseDistDDot=off  SenseIncDDot=off
  footLF : sm_lib/Frames and Transforms/Transform Sensor  MeasurementFrame=World  SenseAngle=off  SenseAxis=off  SenseAngle1=off  SenseAngle2=off  SenseAngle3=off  SenseQ=off  SenseR=off  SenseOmegaX=off  SenseOmegaY=off  SenseOmegaZ=off  SenseOmega1=off  SenseOmega2=off  SenseOmega3=off  SenseQDot=off  SenseRDot=off  SenseAlphaX=off  SenseAlphaY=off  SenseAlphaZ=off  SenseAlpha1=off  SenseAlpha2=off  SenseAlpha3=off  SenseQDDot=off  SenseRDDot=off  SenseX=off  SenseY=off  SenseZ=off  SenseRad=off  SenseAzim=off  SenseDist=off  SenseInc=off  SenseXDot=on  SenseYDot=on  SenseZDot=on  SenseRadDot=off  SenseAzimDot=off  SenseDistDot=off  SenseIncDot=off  SenseXDDot=off  SenseYDDot=off  SenseZDDot=off  SenseRadDDot=off  SenseAzimDDot=off  SenseDistDDot=off  SenseIncDDot=off
  footRB : sm_lib/Frames and Transforms/Transform Sensor  MeasurementFrame=World  SenseAngle=off  SenseAxis=off  SenseAngle1=off  SenseAngle2=off  SenseAngle3=off  SenseQ=off  SenseR=off  SenseOmegaX=off  SenseOmegaY=off  SenseOmegaZ=off  SenseOmega1=off  SenseOmega2=off  SenseOmega3=off  SenseQDot=off  SenseRDot=off  SenseAlphaX=off  SenseAlphaY=off  SenseAlphaZ=off  SenseAlpha1=off  SenseAlpha2=off  SenseAlpha3=off  SenseQDDot=off  SenseRDDot=off  SenseX=off  SenseY=off  SenseZ=off  SenseRad=off  SenseAzim=off  SenseDist=off  SenseInc=off  SenseXDot=on  SenseYDot=on  SenseZDot=on  SenseRadDot=off  SenseAzimDot=off  SenseDistDot=off  SenseIncDot=off  SenseXDDot=off  SenseYDDot=off  SenseZDDot=off  SenseRadDDot=off  SenseAzimDDot=off  SenseDistDDot=off  SenseIncDDot=off
  footRF : sm_lib/Frames and Transforms/Transform Sensor  MeasurementFrame=World  SenseAngle=off  SenseAxis=off  SenseAngle1=off  SenseAngle2=off  SenseAngle3=off  SenseQ=off  SenseR=off  SenseOmegaX=off  SenseOmegaY=off  SenseOmegaZ=off  SenseOmega1=off  SenseOmega2=off  SenseOmega3=off  SenseQDot=off  SenseRDot=off  SenseAlphaX=off  SenseAlphaY=off  SenseAlphaZ=off  SenseAlpha1=off  SenseAlpha2=off  SenseAlpha3=off  SenseQDDot=off  SenseRDDot=off  SenseX=off  SenseY=off  SenseZ=off  SenseRad=off  SenseAzim=off  SenseDist=off  SenseInc=off  SenseXDot=on  SenseYDot=on  SenseZDot=on  SenseRadDot=off  SenseAzimDot=off  SenseDistDot=off  SenseIncDot=off  SenseXDDot=off  SenseYDDot=off  SenseZDDot=off  SenseRadDDot=off  SenseAzimDDot=off  SenseDistDDot=off  SenseIncDDot=off
  lowerlegLB : sm_lib/Frames and Transforms/Transform Sensor  MeasurementFrame=World  SenseAngle=off  SenseAxis=off  SenseAngle1=off  SenseAngle2=off  SenseAngle3=off  SenseQ=off  SenseR=off  SenseOmegaX=off  SenseOmegaY=off  SenseOmegaZ=off  SenseOmega1=off  SenseOmega2=off  SenseOmega3=off  SenseQDot=off  SenseRDot=off  SenseAlphaX=off  SenseAlphaY=off  SenseAlphaZ=off  SenseAlpha1=off  SenseAlpha2=off  SenseAlpha3=off  SenseQDDot=off  SenseRDDot=off  SenseX=off  SenseY=off  SenseZ=off  SenseRad=off  SenseAzim=off  SenseDist=off  SenseInc=off  SenseXDot=on  SenseYDot=on  SenseZDot=on  SenseRadDot=off  SenseAzimDot=off  SenseDistDot=off  SenseIncDot=off  SenseXDDot=off  SenseYDDot=off  SenseZDDot=off  SenseRadDDot=off  SenseAzimDDot=off  SenseDistDDot=off  SenseIncDDot=off
  lowerlegLF : sm_lib/Frames and Transforms/Transform Sensor  MeasurementFrame=World  SenseAngle=off  SenseAxis=off  SenseAngle1=off  SenseAngle2=off  SenseAngle3=off  SenseQ=off  SenseR=off  SenseOmegaX=off  SenseOmegaY=off  SenseOmegaZ=off  SenseOmega1=off  SenseOmega2=off  SenseOmega3=off  SenseQDot=off  SenseRDot=off  SenseAlphaX=off  SenseAlphaY=off  SenseAlphaZ=off  SenseAlpha1=off  SenseAlpha2=off  SenseAlpha3=off  SenseQDDot=off  SenseRDDot=off  SenseX=off  SenseY=off  SenseZ=off  SenseRad=off  SenseAzim=off  SenseDist=off  SenseInc=off  SenseXDot=on  SenseYDot=on  SenseZDot=on  SenseRadDot=off  SenseAzimDot=off  SenseDistDot=off  SenseIncDot=off  SenseXDDot=off  SenseYDDot=off  SenseZDDot=off  SenseRadDDot=off  SenseAzimDDot=off  SenseDistDDot=off  SenseIncDDot=off
  lowerlegRB : sm_lib/Frames and Transforms/Transform Sensor  MeasurementFrame=World  SenseAngle=off  SenseAxis=off  SenseAngle1=off  SenseAngle2=off  SenseAngle3=off  SenseQ=off  SenseR=off  SenseOmegaX=off  SenseOmegaY=off  SenseOmegaZ=off  SenseOmega1=off  SenseOmega2=off  SenseOmega3=off  SenseQDot=off  SenseRDot=off  SenseAlphaX=off  SenseAlphaY=off  SenseAlphaZ=off  SenseAlpha1=off  SenseAlpha2=off  SenseAlpha3=off  SenseQDDot=off  SenseRDDot=off  SenseX=off  SenseY=off  SenseZ=off  SenseRad=off  SenseAzim=off  SenseDist=off  SenseInc=off  SenseXDot=on  SenseYDot=on  SenseZDot=on  SenseRadDot=off  SenseAzimDot=off  SenseDistDot=off  SenseIncDot=off  SenseXDDot=off  SenseYDDot=off  SenseZDDot=off  SenseRadDDot=off  SenseAzimDDot=off  SenseDistDDot=off  SenseIncDDot=off
  lowerlegRF : sm_lib/Frames and Transforms/Transform Sensor  MeasurementFrame=World  SenseAngle=off  SenseAxis=off  SenseAngle1=off  SenseAngle2=off  SenseAngle3=off  SenseQ=off  SenseR=off  SenseOmegaX=off  SenseOmegaY=off  SenseOmegaZ=off  SenseOmega1=off  SenseOmega2=off  SenseOmega3=off  SenseQDot=off  SenseRDot=off  SenseAlphaX=off  SenseAlphaY=off  SenseAlphaZ=off  SenseAlpha1=off  SenseAlpha2=off  SenseAlpha3=off  SenseQDDot=off  SenseRDDot=off  SenseX=off  SenseY=off  SenseZ=off  SenseRad=off  SenseAzim=off  SenseDist=off  SenseInc=off  SenseXDot=on  SenseYDot=on  SenseZDot=on  SenseRadDot=off  SenseAzimDot=off  SenseDistDot=off  SenseIncDot=off  SenseXDDot=off  SenseYDDot=off  SenseZDDot=off  SenseRadDDot=off  SenseAzimDDot=off  SenseDistDDot=off  SenseIncDDot=off
  torso : sm_lib/Frames and Transforms/Transform Sensor  MeasurementFrame=World  SenseAngle=off  SenseAxis=off  SenseAngle1=off  SenseAngle2=off  SenseAngle3=off  SenseQ=off  SenseR=off  SenseOmegaX=off  SenseOmegaY=off  SenseOmegaZ=off  SenseOmega1=off  SenseOmega2=off  SenseOmega3=off  SenseQDot=off  SenseRDot=off  SenseAlphaX=off  SenseAlphaY=off  SenseAlphaZ=off  SenseAlpha1=off  SenseAlpha2=off  SenseAlpha3=off  SenseQDDot=off  SenseRDDot=off  SenseX=off  SenseY=off  SenseZ=off  SenseRad=off  SenseAzim=off  SenseDist=off  SenseInc=off  SenseXDot=on  SenseYDot=on  SenseZDot=on  SenseRadDot=off  SenseAzimDot=off  SenseDistDot=off  SenseIncDot=off  SenseXDDot=off  SenseYDDot=off  SenseZDDot=off  SenseRadDDot=off  SenseAzimDDot=off  SenseDistDDot=off  SenseIncDDot=off
  upperlegLB1 : sm_lib/Frames and Transforms/Transform Sensor  MeasurementFrame=World  SenseAngle=off  SenseAxis=off  SenseAngle1=off  SenseAngle2=off  SenseAngle3=off  SenseQ=off  SenseR=off  SenseOmegaX=off  SenseOmegaY=off  SenseOmegaZ=off  SenseOmega1=off  SenseOmega2=off  SenseOmega3=off  SenseQDot=off  SenseRDot=off  SenseAlphaX=off  SenseAlphaY=off  SenseAlphaZ=off  SenseAlpha1=off  SenseAlpha2=off  SenseAlpha3=off  SenseQDDot=off  SenseRDDot=off  SenseX=off  SenseY=off  SenseZ=off  SenseRad=off  SenseAzim=off  SenseDist=off  SenseInc=off  SenseXDot=on  SenseYDot=on  SenseZDot=on  SenseRadDot=off  SenseAzimDot=off  SenseDistDot=off  SenseIncDot=off  SenseXDDot=off  SenseYDDot=off  SenseZDDot=off  SenseRadDDot=off  SenseAzimDDot=off  SenseDistDDot=off  SenseIncDDot=off
  upperlegLF : sm_lib/Frames and Transforms/Transform Sensor  MeasurementFrame=World  SenseAngle=off  SenseAxis=off  SenseAngle1=off  SenseAngle2=off  SenseAngle3=off  SenseQ=off  SenseR=off  SenseOmegaX=off  SenseOmegaY=off  SenseOmegaZ=off  SenseOmega1=off  SenseOmega2=off  SenseOmega3=off  SenseQDot=off  SenseRDot=off  SenseAlphaX=off  SenseAlphaY=off  SenseAlphaZ=off  SenseAlpha1=off  SenseAlpha2=off  SenseAlpha3=off  SenseQDDot=off  SenseRDDot=off  SenseX=off  SenseY=off  SenseZ=off  SenseRad=off  SenseAzim=off  SenseDist=off  SenseInc=off  SenseXDot=on  SenseYDot=on  SenseZDot=on  SenseRadDot=off  SenseAzimDot=off  SenseDistDot=off  SenseIncDot=off  SenseXDDot=off  SenseYDDot=off  SenseZDDot=off  SenseRadDDot=off  SenseAzimDDot=off  SenseDistDDot=off  SenseIncDDot=off
  upperlegRB : sm_lib/Frames and Transforms/Transform Sensor  MeasurementFrame=World  SenseAngle=off  SenseAxis=off  SenseAngle1=off  SenseAngle2=off  SenseAngle3=off  SenseQ=off  SenseR=off  SenseOmegaX=off  SenseOmegaY=off  SenseOmegaZ=off  SenseOmega1=off  SenseOmega2=off  SenseOmega3=off  SenseQDot=off  SenseRDot=off  SenseAlphaX=off  SenseAlphaY=off  SenseAlphaZ=off  SenseAlpha1=off  SenseAlpha2=off  SenseAlpha3=off  SenseQDDot=off  SenseRDDot=off  SenseX=off  SenseY=off  SenseZ=off  SenseRad=off  SenseAzim=off  SenseDist=off  SenseInc=off  SenseXDot=on  SenseYDot=on  SenseZDot=on  SenseRadDot=off  SenseAzimDot=off  SenseDistDot=off  SenseIncDot=off  SenseXDDot=off  SenseYDDot=off  SenseZDDot=off  SenseRadDDot=off  SenseAzimDDot=off  SenseDistDDot=off  SenseIncDDot=off
  upperlegRF : sm_lib/Frames and Transforms/Transform Sensor  MeasurementFrame=World  SenseAngle=off  SenseAxis=off  SenseAngle1=off  SenseAngle2=off  SenseAngle3=off  SenseQ=off  SenseR=off  SenseOmegaX=off  SenseOmegaY=off  SenseOmegaZ=off  SenseOmega1=off  SenseOmega2=off  SenseOmega3=off  SenseQDot=off  SenseRDot=off  SenseAlphaX=off  SenseAlphaY=off  SenseAlphaZ=off  SenseAlpha1=off  SenseAlpha2=off  SenseAlpha3=off  SenseQDDot=off  SenseRDDot=off  SenseX=off  SenseY=off  SenseZ=off  SenseRad=off  SenseAzim=off  SenseDist=off  SenseInc=off  SenseXDot=on  SenseYDot=on  SenseZDot=on  SenseRadDot=off  SenseAzimDot=off  SenseDistDot=off  SenseIncDot=off  SenseXDDot=off  SenseYDDot=off  SenseZDDot=off  SenseRadDDot=off  SenseAzimDDot=off  SenseDistDDot=off  SenseIncDDot=off
  Conn5 : PMIOPort  Side=Left
  Conn4 : PMIOPort  Port=2  Side=Right
  Conn10 : PMIOPort  Port=3  Side=Right
  Conn11 : PMIOPort  Port=4  Side=Right
  Conn12 : PMIOPort  Port=5  Side=Right
  Conn13 : PMIOPort  Port=6  Side=Right
  Conn14 : PMIOPort  Port=7  Side=Right
  Conn15 : PMIOPort  Port=8  Side=Right
  Conn16 : PMIOPort  Port=9  Side=Right
  Conn17 : PMIOPort  Port=10  Side=Right
  Conn18 : PMIOPort  Port=11  Side=Right
  Conn19 : PMIOPort  Port=12  Side=Right
  Conn20 : PMIOPort  Port=13  Side=Right
  Conn21 : PMIOPort  Port=14  Side=Right
  Outport : Outport
  wires:
  PS-Simulink Converter10/1 -> MATLAB Function7/2(vy)
  PS-Simulink Converter13/1 -> MATLAB Function2/1(vx)
  MATLAB Function12/1(v) -> MATLAB Function13/10(vulLB)
  PS-Simulink Converter36/1 -> MATLAB Function12/3(vz)
  PS-Simulink Converter14/1 -> MATLAB Function2/2(vy)
  PS-Simulink Converter9/1 -> MATLAB Function7/1(vx)
  PS-Simulink Converter11/1 -> MATLAB Function7/3(vz)
  PS-Simulink Converter8/1 -> MATLAB Function1/2(vy)
  PS-Simulink Converter7/1 -> MATLAB Function6/3(vz)
  PS-Simulink Converter38/1 -> MATLAB Function5/2(vy)
  PS-Simulink Converter16/1 -> MATLAB Function3/1(vx)
  MATLAB Function9/1(v) -> MATLAB Function13/11(vllLB)
  MATLAB Function1/1(v) -> MATLAB Function13/1(vulRF)
  PS-Simulink Converter17/1 -> MATLAB Function3/2(vy)
  PS-Simulink Converter28/1 -> MATLAB Function10/1(vx)
  PS-Simulink Converter21/1 -> MATLAB Function4/3(vz)
  PS-Simulink Converter18/1 -> MATLAB Function3/3(vz)
  PS-Simulink Converter6/1 -> MATLAB Function1/1(vx)
  PS-Simulink Converter19/1 -> MATLAB Function4/1(vx)
  PS-Simulink Converter5/1 -> MATLAB Function6/2(vy)
  PS-Simulink Converter20/1 -> MATLAB Function4/2(vy)
  PS-Simulink Converter12/1 -> MATLAB Function1/3(vz)
  PS-Simulink Converter15/1 -> MATLAB Function2/3(vz)
  PS-Simulink Converter39/1 -> MATLAB Function5/3(vz)
  MATLAB Function2/1(v) -> MATLAB Function13/2(vllRF)
  MATLAB Function10/1(v) -> MATLAB Function13/12(vfLB)
  PS-Simulink Converter27/1 -> MATLAB Function9/3(vz)
  PS-Simulink Converter4/1 -> MATLAB Function6/1(vx)
  PS-Simulink Converter25/1 -> MATLAB Function9/1(vx)
  PS-Simulink Converter37/1 -> MATLAB Function5/1(vx)
  PS-Simulink Converter26/1 -> MATLAB Function9/2(vy)
  PS-Simulink Converter24/1 -> MATLAB Function8/3(vz)
  PS-Simulink Converter22/1 -> MATLAB Function8/1(vx)
  PS-Simulink Converter23/1 -> MATLAB Function8/2(vy)
  PS-Simulink Converter34/1 -> MATLAB Function12/1(vx)
  PS-Simulink Converter35/1 -> MATLAB Function12/2(vy)
  MATLAB Function7/1(v) -> MATLAB Function13/9(vfRB)
  MATLAB Function6/1(v) -> MATLAB Function13/8(vllRB)
  MATLAB Function5/1(v) -> MATLAB Function13/7(vulRB)
  MATLAB Function11/1(v) -> MATLAB Function13/6(vfLF)
  PS-Simulink Converter33/1 -> MATLAB Function11/3(vz)
  MATLAB Function8/1(v) -> MATLAB Function13/5(vllLF)
  MATLAB Function4/1(v) -> MATLAB Function13/4(vulLF)
  MATLAB Function3/1(v) -> MATLAB Function13/3(vfRF)
  PS-Simulink Converter32/1 -> MATLAB Function11/2(vy)
  PS-Simulink Converter31/1 -> MATLAB Function11/1(vx)
  PS-Simulink Converter30/1 -> MATLAB Function10/3(vz)
  PS-Simulink Converter29/1 -> MATLAB Function10/2(vy)
  PS-Simulink Converter3/1 -> MATLAB Function14/1(vx)
  PS-Simulink Converter1/1 -> MATLAB Function14/2(vy)
  PS-Simulink Converter2/1 -> MATLAB Function14/3(vz)
  MATLAB Function14/1(v) -> MATLAB Function13/13(v_torso)
  MATLAB Function13/1(Mvcm) -> Outport/1
  connections:
  footRB/RConn4 -- PS-Simulink Converter11/LConn1
  lowerlegLF/RConn2 -- PS-Simulink Converter22/LConn1
  upperlegLF/RConn4 -- PS-Simulink Converter21/LConn1
  footLB/RConn2 -- PS-Simulink Converter28/LConn1
  upperlegLB1/RConn1 -- Conn19/RConn1
  footLF/RConn2 -- PS-Simulink Converter31/LConn1
  lowerlegLB/LConn1 -- upperlegLB1/LConn1 -- footRB/LConn1 -- upperlegLF/LConn1 -- lowerlegRF/LConn1 -- upperlegRF/LConn1 -- footRF/LConn1 -- lowerlegLF/LConn1 -- footLF/LConn1 -- Conn5/RConn1 -- torso/LConn1 -- upperlegRB/LConn1 -- lowerlegRB/LConn1 -- footLB/LConn1
  lowerlegRB/RConn4 -- PS-Simulink Converter7/LConn1
  Conn17/RConn1 -- lowerlegRB/RConn1
  upperlegLF/RConn2 -- PS-Simulink Converter19/LConn1
  upperlegLF/RConn3 -- PS-Simulink Converter20/LConn1
  lowerlegRF/RConn3 -- PS-Simulink Converter14/LConn1
  footLB/RConn4 -- PS-Simulink Converter30/LConn1
  footRB/RConn3 -- PS-Simulink Converter10/LConn1
  upperlegRB/RConn3 -- PS-Simulink Converter38/LConn1
  lowerlegRF/RConn2 -- PS-Simulink Converter13/LConn1
  upperlegRB/RConn4 -- PS-Simulink Converter39/LConn1
  upperlegRB/RConn2 -- PS-Simulink Converter37/LConn1
  upperlegRF/RConn2 -- PS-Simulink Converter6/LConn1
  footLB/RConn1 -- Conn21/RConn1
  lowerlegRF/RConn4 -- PS-Simulink Converter15/LConn1
  lowerlegLF/RConn4 -- PS-Simulink Converter24/LConn1
  upperlegLB1/RConn4 -- PS-Simulink Converter36/LConn1
  PS-Simulink Converter16/LConn1 -- footRF/RConn2
  footRB/RConn2 -- PS-Simulink Converter9/LConn1
  footRF/RConn3 -- PS-Simulink Converter17/LConn1
  footRF/RConn4 -- PS-Simulink Converter18/LConn1
  upperlegRF/RConn4 -- PS-Simulink Converter12/LConn1
  upperlegRF/RConn3 -- PS-Simulink Converter8/LConn1
  lowerlegLF/RConn3 -- PS-Simulink Converter23/LConn1
  lowerlegRB/RConn3 -- PS-Simulink Converter5/LConn1
  lowerlegRB/RConn2 -- PS-Simulink Converter4/LConn1
  lowerlegLB/RConn3 -- PS-Simulink Converter26/LConn1
  lowerlegLB/RConn4 -- PS-Simulink Converter27/LConn1
  lowerlegLB/RConn2 -- PS-Simulink Converter25/LConn1
  lowerlegLB/RConn1 -- Conn20/RConn1
  upperlegLB1/RConn3 -- PS-Simulink Converter35/LConn1
  upperlegLB1/RConn2 -- PS-Simulink Converter34/LConn1
  upperlegRF/RConn1 -- Conn10/RConn1
  upperlegLF/RConn1 -- Conn13/RConn1
  footLF/RConn3 -- PS-Simulink Converter32/LConn1
  footLF/RConn4 -- PS-Simulink Converter33/LConn1
  footLB/RConn3 -- PS-Simulink Converter29/LConn1
  Conn18/RConn1 -- footRB/RConn1
  footLF/RConn1 -- Conn15/RConn1
  Conn16/RConn1 -- upperlegRB/RConn1
  lowerlegLF/RConn1 -- Conn14/RConn1
  Conn11/RConn1 -- lowerlegRF/RConn1
  footRF/RConn1 -- Conn12/RConn1
  torso/RConn1 -- Conn4/RConn1
  torso/RConn3 -- PS-Simulink Converter1/LConn1
  torso/RConn2 -- PS-Simulink Converter3/LConn1
  torso/RConn4 -- PS-Simulink Converter2/LConn1
